simulink model "Controlador_PID"  (R2023b)
settings: Solver=ode1  StartTime=0.0  StopTime=10.0  FixedStep=0.01  RelTol=1e-3
settings Model: Creator=Nacho Andrade  LastModifiedBy=Nacho Andrade

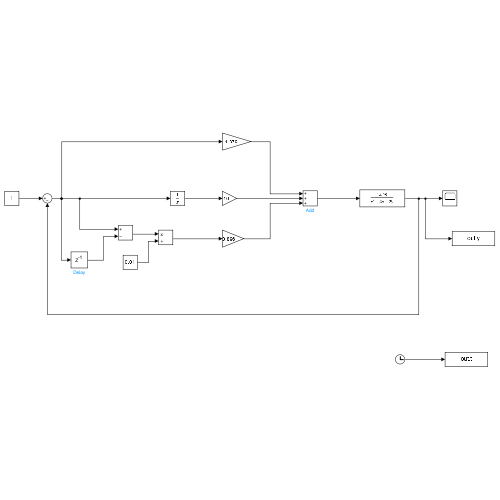
[thumbnail: Simulink's stored preview of the top-level diagram]
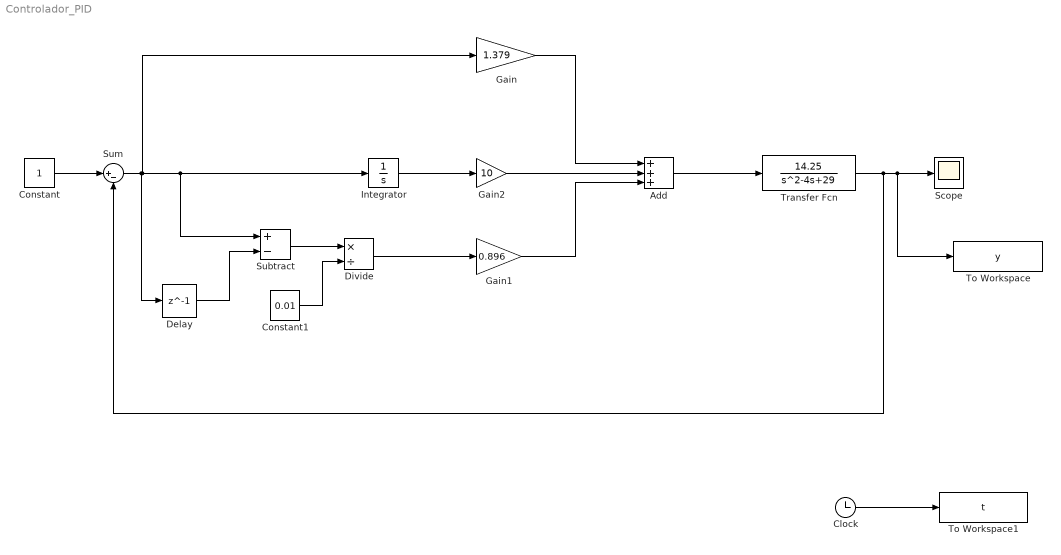
== system Controlador_PID ==
  Add : Sum  Inputs=+++
  Clock : Clock
  Constant : Constant
  Constant1 : Constant  Value=0.01
  Delay : Delay  DelayLength=1
  Divide : Product  Inputs=*/
  Gain : Gain  Gain=1.379
  Gain1 : Gain  Gain=0.896
  Gain2 : Gain  Gain=10
  Integrator : Integrator
  Scope : Scope
  Subtract : Sum  Inputs=+-
  Sum : Sum  Inputs=|+-
  To Workspace : ToWorkspace  VariableName=y  SampleTime=-1
  To Workspace1 : ToWorkspace  VariableName=t  SampleTime=-1
  Transfer Fcn : TransferFcn  Numerator=[14.25]  Denominator=[1 -4 29]
  wires:
  Constant/1 -> Sum/1
  Integrator/1 -> Gain2/1
  Sum/1 -> Delay/1, Gain/1, Subtract/1, Integrator/1
  Delay/1 -> Subtract/2
  Subtract/1 -> Divide/1
  Constant1/1 -> Divide/2
  Divide/1 -> Gain1/1
  Gain2/1 -> Add/2
  Gain/1 -> Add/1
  Gain1/1 -> Add/3
  Transfer Fcn/1 -> Sum/2, To Workspace/1, Scope/1
  Add/1 -> Transfer Fcn/1
  Clock/1 -> To Workspace1/1
